simulink model "Adaptive"  (R2016b)
settings: Solver=VariableStepAuto  StartTime=0.0  StopTime=40  FixedStep=Ts  RelTol=1e-3
values from neighbouring files (symbols this model uses):
  A = [0 1;0 0]    [Adaptive.m]
  Am = [-2*xim*wm -wm^2;1 0]    [Adaptive.m]
  B = [0;K]    [Adaptive.m]
  Bm = [1;0]    [Adaptive.m]
  C = [1 0]    [Adaptive.m]
  Cm = [0 wm^2]    [Adaptive.m]
  D = 0    [Adaptive.m]
  Dm = 0    [Adaptive.m]
  down = -up    (= -0.0872664625997)    [Adaptive.m]
  gammar = 1    [Adaptive.m]
  gammax = diag([35 10])    [Adaptive.m]
  P_bar = [double(S.p12);double(S.p22)]    [Adaptive.m]
  up = 5*pi/180    (= 0.0872664625997)    [Adaptive.m]
settings Model: Creator=Ashraf  LastModifiedBy=Ashraf

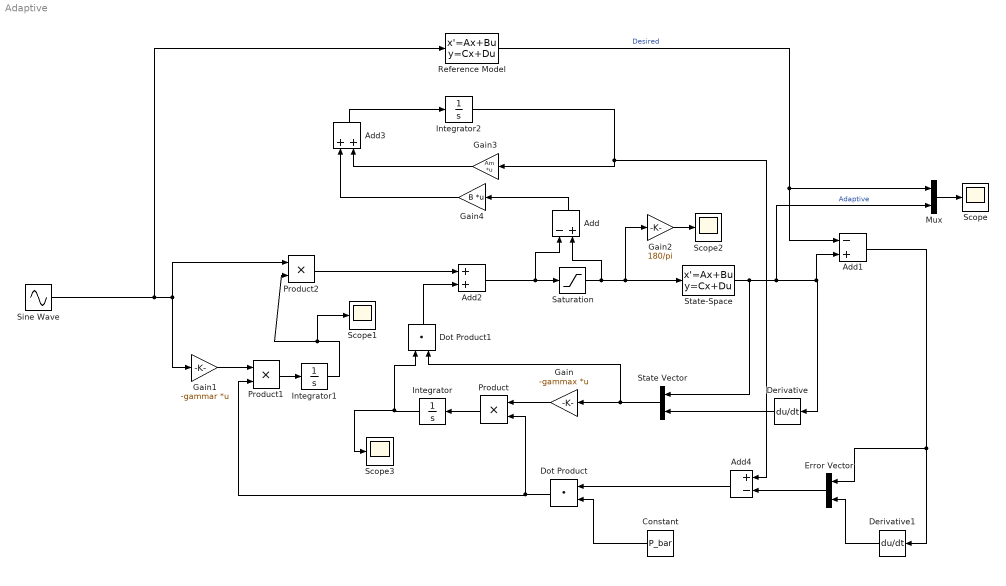
== system Adaptive ==
  Add : Sum  Inputs=-+
  Add1 : Sum  Inputs=-+
  Add2 : Sum
  Add3 : Sum
  Add4 : Sum  Inputs=+-
  Constant : Constant  Value=P_bar
  Derivative : Derivative
  Derivative1 : Derivative
  Dot Product : DotProduct  InputSameDT=on  OutDataTypeStr=Inherit: Inherit via internal rule
  Dot Product1 : DotProduct  InputSameDT=on  OutDataTypeStr=Inherit: Inherit via internal rule
  Error Vector : Concatenate
  Gain : Gain  Gain=-gammax  Multiplication=Matrix(K*u)
  Gain1 : Gain  Gain=-gammar  Multiplication=Matrix(K*u)
  Gain2 : Gain  Gain=180/pi
  Gain3 : Gain  Gain=Am  Multiplication=Matrix(K*u)
  Gain4 : Gain  Gain=B  Multiplication=Matrix(K*u)
  Integrator : Integrator
  Integrator1 : Integrator
  Integrator2 : Integrator
  Mux : Mux  Inputs=2
  Product : Product
  Product1 : Product
  Product2 : Product
  Reference Model : StateSpace  A=Am  B=Bm  C=Cm  D=Dm  X0=[0 0]
  Saturation : Saturate  UpperLimit=up  LowerLimit=down
  Scope{,1..3} (4 alike) : Scope
  Sine Wave : Sin  Amplitude=0.2  SampleTime=0
  State Vector : Concatenate
  State-Space : StateSpace  A=A  B=B  C=C  D=D  X0=[0 0]
  wires:
  State-Space/1 -> Mux/2, Add1/2, Derivative/1, State Vector/1  "Adaptive"
  Sine Wave/1 -> Gain1/1, Product2/1, Reference Model/1
  Reference Model/1 -> Mux/1, Add1/1  "Desired"
  Add1/1 -> Derivative1/1, Error Vector/1
  Derivative1/1 -> Error Vector/2
  Constant/1 -> Dot Product/2
  Derivative/1 -> State Vector/2
  State Vector/1 -> Dot Product1/2, Gain/1
  Dot Product/1 -> Product/2, Product1/2
  Gain/1 -> Product/1
  Product/1 -> Integrator/1
  Integrator/1 -> Scope3/1, Dot Product1/1
  Gain1/1 -> Product1/1
  Product1/1 -> Integrator1/1
  Integrator1/1 -> Scope1/1, Product2/2
  Product2/1 -> Add2/1
  Dot Product1/1 -> Add2/2
  Gain2/1 -> Scope2/1
  Add2/1 -> Add/1, Saturation/1
  Mux/1 -> Scope/1
  Saturation/1 -> Add/2, State-Space/1, Gain2/1
  Add/1 -> Gain4/1
  Gain3/1 -> Add3/2
  Gain4/1 -> Add3/1
  Add3/1 -> Integrator2/1
  Error Vector/1 -> Add4/2
  Integrator2/1 -> Add4/1, Gain3/1
  Add4/1 -> Dot Product/1
